simulink model "PID_MOJ"  (R2022b)
settings: Solver=VariableStepAuto  StartTime=0.0  StopTime=10  RelTol=10e-10
values from neighbouring files (symbols this model uses):
  B = 5    [DANE_TRANSMITANCJA.m]
  D = 1    [DANE_TRANSMITANCJA.m]
  g = 9.81    [DANE_TRANSMITANCJA.m]
  J = 0.2    [DANE_TRANSMITANCJA.m]
  k = 700000    [DANE_TRANSMITANCJA.m]
  ke = 2    [DANE_TRANSMITANCJA.m]
  km = 5    [DANE_TRANSMITANCJA.m]
  Kp = 0.6*Kkr*(1-Tp/Tosc)    (= 22.6944444444)    [DANE_TRANSMITANCJA.m]
  L = 0.1    [DANE_TRANSMITANCJA.m]
  m = 100    [DANE_TRANSMITANCJA.m]
  mp = 100    [DANE_TRANSMITANCJA.m]
  r = 0.2    [DANE_TRANSMITANCJA.m]
  R = 0.4    [DANE_TRANSMITANCJA.m]
  Td = Tp*0.125*(Tosc/Tp)^2/(Tosc/Tp-1)    (= 0.271255813953)    [DANE_TRANSMITANCJA.m]
  Ti = Tp*0.5*(Tosc/Tp-1)    (= 1.075)    [DANE_TRANSMITANCJA.m]
  Tp = 0.01    [DANE_TRANSMITANCJA.m]
undefined symbols (not defined in the file or in its folder): Ld, Md
libraries: slpidlib x4, fuzblock x1
settings Model: Creator=ThePi  LastModifiedBy=ThePi

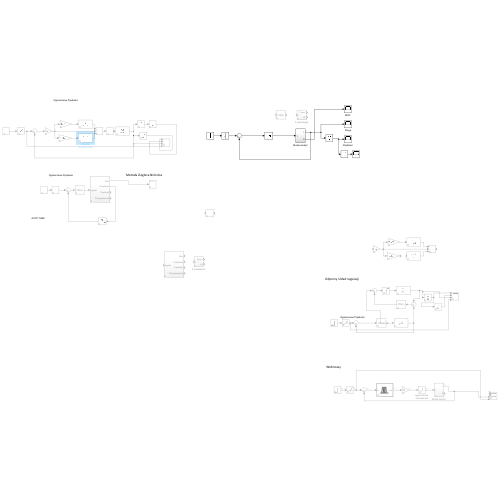
[thumbnail: Simulink's stored preview of the top-level diagram]
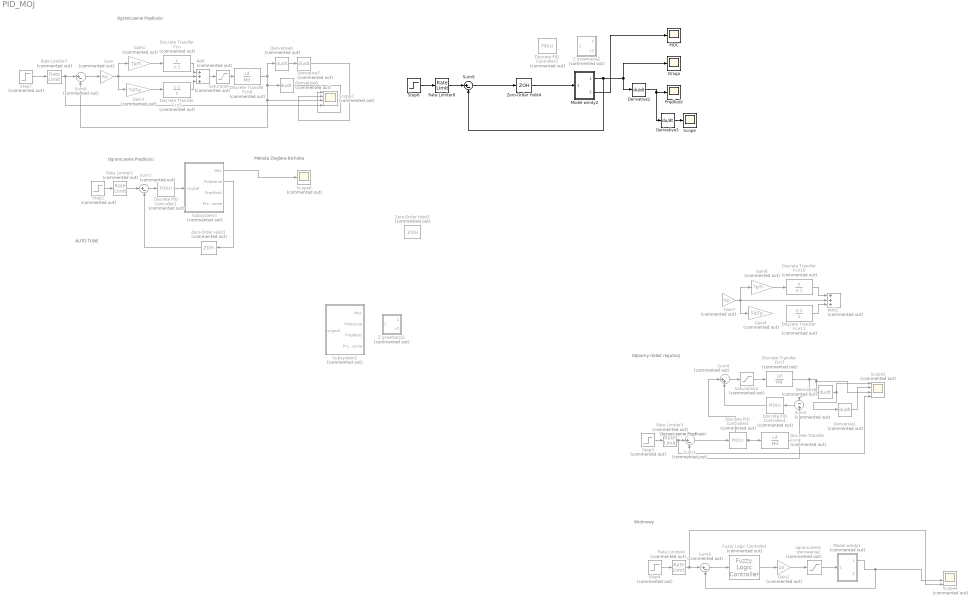
== system PID_MOJ ==
  note: Ograniczenie Prędkości
  note: Metoda Zieglera-Nicholsa
  note: AUTO TUNE
  note: Odporny Układ regulacji
  note: Ograniczenie Prędkości
  note: Ograniczenie Prędkości
  note: WIdmowy
  Add : Sum  Commented=on  Inputs=+++
  Add2 : Sum  Commented=on  Inputs=+++
  Derivative{,1,6..8} (5 alike) : Derivative  Commented=on
  Derivative2 : Derivative
  Derivative3 : Derivative
  Discrete Transfer Fcn : DiscreteTransferFcn  Commented=on  Numerator=[1 0]  Denominator=[1 -1]
  Discrete Transfer Fcn10 : DiscreteTransferFcn  Commented=on  Numerator=[1 0]  Denominator=[1 -1]
  Discrete Transfer Fcn11 : DiscreteTransferFcn  Commented=on  Numerator=[1 -1]  Denominator=[1 0]
  Discrete Transfer Fcn4 : DiscreteTransferFcn  Commented=on  Numerator=Ld  Denominator=Md  SampleTime=Tp
  Discrete Transfer Fcn5 : DiscreteTransferFcn  Commented=on  Numerator=[1 -1]  Denominator=[1 0]
  Discrete Transfer Fcn7 : DiscreteTransferFcn  Commented=on  Numerator=Ld  Denominator=Md  SampleTime=Tp
  Discrete Transfer Fcn8 : DiscreteTransferFcn  Commented=on  Numerator=Ld  Denominator=Md  SampleTime=Tp
  Discrete PID Controller1 : slpidlib/PID Controller  Commented=on  Controller=PID  Form=Ideal  TimeDomain=Discrete-time  UseExternalTs=off  SampleTime=Tp  IntegratorMethod=Forward Euler  FilterMethod=Forward Euler  ControllerParametersSource=internal  P=Kp  I=Ti  UseKiTs=off  D=Td  N=182.532020744323  UseFilter=off  TunerSelectOption=Transfer Function Based (PID Tuner App)  InitialConditionSource=internal  InitialConditionForIntegrator=0  InitialConditionForFilter=0  DifferentiatorICPrevScaledInput=0  ExternalReset=none  TrackingMode=off  Kt=1  LimitOutput=off  SatLimitsSource=internal  UpperSaturationLimit=inf  LowerSaturationLimit=-inf  LinearizeAsGain=off  AntiWindupMode=none  Kb=1  LimitIntegrator=off  UpperIntegratorSaturationLimit=inf  LowerIntegratorSaturationLimit=-inf  POutMin=[]  POutMax=[]  IOutMin=[]  IOutMax=[]  DOutMin=[]  DOutMax=[]  NOutMin=[]  NOutMax=[]  SumOutMin=[]  SumOutMax=[]  SaturationOutMin=[]  SaturationOutMax=[]  PParamMin=[]  PParamMax=[]  IParamMin=[]  IParamMax=[]  DParamMin=[]  DParamMax=[]  NParamMin=[]  NParamMax=[]  KbParamMin=[]  KbParamMax=[]  KtParamMin=[]  KtParamMax=[]  KbOutMin=[]  KbOutMax=[]  KtOutMin=[]  KtOutMax=[]  IntegratorOutMin=[]  IntegratorOutMax=[]  FilterOutMin=[]  FilterOutMax=[]  SumI1OutMin=[]  SumI1OutMax=[]  SumI2OutMin=[]  SumI2OutMax=[]  SumI3OutMin=[]  SumI3OutMax=[]  SumI4OutMin=[]  SumI4OutMax=[]  SumDOutMin=[]  SumDOutMax=[]  DifferentiatorOutMin=[]  DifferentiatorOutMax=[]  FilterDiffOutCoefMin=[]  FilterDiffOutCoefMax=[]  ReciprocalOutMin=[]  ReciprocalOutMax=[]  SumDenOutMin=[]  SumDenOutMax=[]  SumNumOutMin=[]  SumNumOutMax=[]  DivideOutMin=[]  DivideOutMax=[]  UdiffTsProdOutMin=[]  UdiffTsProdOutMax=[]  NTsProdOutMin=[]  NTsProdOutMax=[]  UintegralTsProdOutMin=[]  UintegralTsProdOutMax=[]  UngainTsProdOutMin=[]  UngainTsProdOutMax=[]  ClampingZeroOutDataTypeStr=Inherit: Inherit via back propagation  ClampingZeroOutMin=[]  ClampingZeroOutMax=[]  FilterDenConstantOutDataTypeStr=Inherit: Inherit via back propagation  FilterDenConstantOutMin=[]  FilterDenConstantOutMax=[]  PCopyOutDataTypeStr=Inherit: Inherit via back propagation  PCopyOutMin=[]  PCopyOutMax=[]  NCopyOutDataTypeStr=Inherit: Inherit via back propagation  NCopyOutMin=[]  NCopyOutMax=[]  IntegratorContinuousStateAttributes=''  IntegratorStateMustResolveToSignalObject=off  IntegratorRTWStateStorageClass=Auto  FilterContinuousStateAttributes=''  FilterStateMustResolveToSignalObject=off  FilterRTWStateStorageClass=Auto  ParallelPVariant=Passthrough  IdealPVariant=InternalParameters  IVariant=InternalParameters  DVariant=InternalParameters  IntegratorVariant=Discrete  SatVariant=Disabled  AWVariant=Passthrough  PCopyVariant=Disabled  TRVariant=Disabled  FdbkBlocksVariant=Forward  IdealPFdbkVariant=Disabled  SatFdbkVariant=Disabled  DerivativeFilterVariant=Differentiator  NVariant=Passthrough  NCopyVariant=Disabled_SignalSpec  FilterICVariant=InternalICsDifferentiator  IntegratorICVariant=InternalICs  ExternalResetVariant=Disabled  TRSumVariant=Passthrough  SumFdbkVariant=Disabled  SumVariant=Sum_PID  TsampFilterVariant=InternalTs  TsampNgainVariant=Passthrough  TsampIntegralVariant=Passthrough  ExternalSaturationOutDataTypeStr=Inherit: Same as second input
      settings: LibrarySourceBlock=simulink/Discrete/Discrete PID Controller
  Discrete PID Controller2 : slpidlib/PID Controller  Commented=on  Controller=PID  Form=Ideal  TimeDomain=Discrete-time  UseExternalTs=off  SampleTime=Tp  IntegratorMethod=Forward Euler  FilterMethod=Forward Euler  ControllerParametersSource=internal  P=0.623272871396858  I=0.0120978996964584  UseKiTs=off  D=8.78542633879277  N=15.243341638906  UseFilter=on  TunerSelectOption=Transfer Function Based (PID Tuner App)  InitialConditionSource=internal  InitialConditionForIntegrator=0  InitialConditionForFilter=0  DifferentiatorICPrevScaledInput=0  ExternalReset=none  TrackingMode=off  Kt=1  LimitOutput=off  SatLimitsSource=internal  UpperSaturationLimit=inf  LowerSaturationLimit=-inf  LinearizeAsGain=off  AntiWindupMode=none  Kb=1  LimitIntegrator=off  UpperIntegratorSaturationLimit=inf  LowerIntegratorSaturationLimit=-inf  POutMin=[]  POutMax=[]  IOutMin=[]  IOutMax=[]  DOutMin=[]  DOutMax=[]  NOutMin=[]  NOutMax=[]  SumOutMin=[]  SumOutMax=[]  SaturationOutMin=[]  SaturationOutMax=[]  PParamMin=[]  PParamMax=[]  IParamMin=[]  IParamMax=[]  DParamMin=[]  DParamMax=[]  NParamMin=[]  NParamMax=[]  KbParamMin=[]  KbParamMax=[]  KtParamMin=[]  KtParamMax=[]  KbOutMin=[]  KbOutMax=[]  KtOutMin=[]  KtOutMax=[]  IntegratorOutMin=[]  IntegratorOutMax=[]  FilterOutMin=[]  FilterOutMax=[]  SumI1OutMin=[]  SumI1OutMax=[]  SumI2OutMin=[]  SumI2OutMax=[]  SumI3OutMin=[]  SumI3OutMax=[]  SumI4OutMin=[]  SumI4OutMax=[]  SumDOutMin=[]  SumDOutMax=[]  DifferentiatorOutMin=[]  DifferentiatorOutMax=[]  FilterDiffOutCoefMin=[]  FilterDiffOutCoefMax=[]  ReciprocalOutMin=[]  ReciprocalOutMax=[]  SumDenOutMin=[]  SumDenOutMax=[]  SumNumOutMin=[]  SumNumOutMax=[]  DivideOutMin=[]  DivideOutMax=[]  UdiffTsProdOutMin=[]  UdiffTsProdOutMax=[]  NTsProdOutMin=[]  NTsProdOutMax=[]  UintegralTsProdOutMin=[]  UintegralTsProdOutMax=[]  UngainTsProdOutMin=[]  UngainTsProdOutMax=[]  ClampingZeroOutDataTypeStr=Inherit: Inherit via back propagation  ClampingZeroOutMin=[]  ClampingZeroOutMax=[]  FilterDenConstantOutDataTypeStr=Inherit: Inherit via back propagation  FilterDenConstantOutMin=[]  FilterDenConstantOutMax=[]  PCopyOutDataTypeStr=Inherit: Inherit via back propagation  PCopyOutMin=[]  PCopyOutMax=[]  NCopyOutDataTypeStr=Inherit: Inherit via back propagation  NCopyOutMin=[]  NCopyOutMax=[]  IntegratorContinuousStateAttributes=''  IntegratorStateMustResolveToSignalObject=off  IntegratorRTWStateStorageClass=Auto  FilterContinuousStateAttributes=''  FilterStateMustResolveToSignalObject=off  FilterRTWStateStorageClass=Auto  ParallelPVariant=Passthrough  IdealPVariant=InternalParameters  IVariant=InternalParameters  DVariant=InternalParameters  IntegratorVariant=Discrete  SatVariant=Disabled  AWVariant=Passthrough  PCopyVariant=Disabled  TRVariant=Disabled  FdbkBlocksVariant=Forward  IdealPFdbkVariant=Disabled  SatFdbkVariant=Disabled  DerivativeFilterVariant=ForwardEulerFilter  NVariant=InternalParameters  NCopyVariant=Disabled  FilterICVariant=InternalICsFilter  IntegratorICVariant=InternalICs  ExternalResetVariant=Disabled  TRSumVariant=Passthrough  SumFdbkVariant=Disabled  SumVariant=Sum_PID  TsampFilterVariant=InternalTs  TsampNgainVariant=Passthrough  TsampIntegralVariant=Passthrough  ExternalSaturationOutDataTypeStr=Inherit: Same as second input
      settings: LibrarySourceBlock=simulink/Discrete/Discrete PID Controller
  Discrete PID Controller4 : slpidlib/PID Controller  Commented=on  Controller=PID  Form=Parallel  TimeDomain=Discrete-time  UseExternalTs=off  SampleTime=-1  IntegratorMethod=Forward Euler  FilterMethod=Forward Euler  ControllerParametersSource=internal  P=19.8736932517728  I=4.86889756951287  UseKiTs=off  D=6.56817655006432  N=182.532020744323  UseFilter=off  TunerSelectOption=Transfer Function Based (PID Tuner App)  InitialConditionSource=internal  InitialConditionForIntegrator=0  InitialConditionForFilter=0  DifferentiatorICPrevScaledInput=0  ExternalReset=none  TrackingMode=off  Kt=1  LimitOutput=off  SatLimitsSource=internal  UpperSaturationLimit=inf  LowerSaturationLimit=-inf  LinearizeAsGain=off  AntiWindupMode=none  Kb=1  LimitIntegrator=off  UpperIntegratorSaturationLimit=inf  LowerIntegratorSaturationLimit=-inf  POutMin=[]  POutMax=[]  IOutMin=[]  IOutMax=[]  DOutMin=[]  DOutMax=[]  NOutMin=[]  NOutMax=[]  SumOutMin=[]  SumOutMax=[]  SaturationOutMin=[]  SaturationOutMax=[]  PParamMin=[]  PParamMax=[]  IParamMin=[]  IParamMax=[]  DParamMin=[]  DParamMax=[]  NParamMin=[]  NParamMax=[]  KbParamMin=[]  KbParamMax=[]  KtParamMin=[]  KtParamMax=[]  KbOutMin=[]  KbOutMax=[]  KtOutMin=[]  KtOutMax=[]  IntegratorOutMin=[]  IntegratorOutMax=[]  FilterOutMin=[]  FilterOutMax=[]  SumI1OutMin=[]  SumI1OutMax=[]  SumI2OutMin=[]  SumI2OutMax=[]  SumI3OutMin=[]  SumI3OutMax=[]  SumI4OutMin=[]  SumI4OutMax=[]  SumDOutMin=[]  SumDOutMax=[]  DifferentiatorOutMin=[]  DifferentiatorOutMax=[]  FilterDiffOutCoefMin=[]  FilterDiffOutCoefMax=[]  ReciprocalOutMin=[]  ReciprocalOutMax=[]  SumDenOutMin=[]  SumDenOutMax=[]  SumNumOutMin=[]  SumNumOutMax=[]  DivideOutMin=[]  DivideOutMax=[]  UdiffTsProdOutMin=[]  UdiffTsProdOutMax=[]  NTsProdOutMin=[]  NTsProdOutMax=[]  UintegralTsProdOutMin=[]  UintegralTsProdOutMax=[]  UngainTsProdOutMin=[]  UngainTsProdOutMax=[]  ClampingZeroOutDataTypeStr=Inherit: Inherit via back propagation  ClampingZeroOutMin=[]  ClampingZeroOutMax=[]  FilterDenConstantOutDataTypeStr=Inherit: Inherit via back propagation  FilterDenConstantOutMin=[]  FilterDenConstantOutMax=[]  PCopyOutDataTypeStr=Inherit: Inherit via back propagation  PCopyOutMin=[]  PCopyOutMax=[]  NCopyOutDataTypeStr=Inherit: Inherit via back propagation  NCopyOutMin=[]  NCopyOutMax=[]  IntegratorContinuousStateAttributes=''  IntegratorStateMustResolveToSignalObject=off  IntegratorRTWStateStorageClass=Auto  FilterContinuousStateAttributes=''  FilterStateMustResolveToSignalObject=off  FilterRTWStateStorageClass=Auto  ParallelPVariant=InternalParameters  IdealPVariant=Disabled  IVariant=InternalParameters  DVariant=InternalParameters  IntegratorVariant=Discrete  SatVariant=Disabled  AWVariant=Passthrough  PCopyVariant=Disabled  TRVariant=Disabled  FdbkBlocksVariant=Forward  IdealPFdbkVariant=Disabled  SatFdbkVariant=Disabled  DerivativeFilterVariant=Differentiator  NVariant=Passthrough  NCopyVariant=Disabled_SignalSpec  FilterICVariant=InternalICsDifferentiator  IntegratorICVariant=InternalICs  ExternalResetVariant=Disabled  TRSumVariant=Passthrough  SumFdbkVariant=Disabled  SumVariant=Sum_PID  TsampFilterVariant=InternalTs  TsampNgainVariant=Passthrough  TsampIntegralVariant=Passthrough  ExternalSaturationOutDataTypeStr=Inherit: Same as second input
      settings: LibrarySourceBlock=simulink/Discrete/Discrete PID Controller
  Discrete PID Controller5 : slpidlib/PID Controller  Commented=on  Controller=PID  Form=Ideal  TimeDomain=Discrete-time  UseExternalTs=off  SampleTime=Tp  IntegratorMethod=Forward Euler  FilterMethod=Forward Euler  ControllerParametersSource=internal  P=18.4427572090829  I=0.268340065032812  UseKiTs=off  D=0.559716120813621  N=30.7688755395407  UseFilter=on  TunerSelectOption=Transfer Function Based (PID Tuner App)  InitialConditionSource=internal  InitialConditionForIntegrator=0  InitialConditionForFilter=0  DifferentiatorICPrevScaledInput=0  ExternalReset=none  TrackingMode=off  Kt=1  LimitOutput=off  SatLimitsSource=internal  UpperSaturationLimit=inf  LowerSaturationLimit=-inf  LinearizeAsGain=off  AntiWindupMode=none  Kb=1  LimitIntegrator=off  UpperIntegratorSaturationLimit=inf  LowerIntegratorSaturationLimit=-inf  POutMin=[]  POutMax=[]  IOutMin=[]  IOutMax=[]  DOutMin=[]  DOutMax=[]  NOutMin=[]  NOutMax=[]  SumOutMin=[]  SumOutMax=[]  SaturationOutMin=[]  SaturationOutMax=[]  PParamMin=[]  PParamMax=[]  IParamMin=[]  IParamMax=[]  DParamMin=[]  DParamMax=[]  NParamMin=[]  NParamMax=[]  KbParamMin=[]  KbParamMax=[]  KtParamMin=[]  KtParamMax=[]  KbOutMin=[]  KbOutMax=[]  KtOutMin=[]  KtOutMax=[]  IntegratorOutMin=[]  IntegratorOutMax=[]  FilterOutMin=[]  FilterOutMax=[]  SumI1OutMin=[]  SumI1OutMax=[]  SumI2OutMin=[]  SumI2OutMax=[]  SumI3OutMin=[]  SumI3OutMax=[]  SumI4OutMin=[]  SumI4OutMax=[]  SumDOutMin=[]  SumDOutMax=[]  DifferentiatorOutMin=[]  DifferentiatorOutMax=[]  FilterDiffOutCoefMin=[]  FilterDiffOutCoefMax=[]  ReciprocalOutMin=[]  ReciprocalOutMax=[]  SumDenOutMin=[]  SumDenOutMax=[]  SumNumOutMin=[]  SumNumOutMax=[]  DivideOutMin=[]  DivideOutMax=[]  UdiffTsProdOutMin=[]  UdiffTsProdOutMax=[]  NTsProdOutMin=[]  NTsProdOutMax=[]  UintegralTsProdOutMin=[]  UintegralTsProdOutMax=[]  UngainTsProdOutMin=[]  UngainTsProdOutMax=[]  ClampingZeroOutDataTypeStr=Inherit: Inherit via back propagation  ClampingZeroOutMin=[]  ClampingZeroOutMax=[]  FilterDenConstantOutDataTypeStr=Inherit: Inherit via back propagation  FilterDenConstantOutMin=[]  FilterDenConstantOutMax=[]  PCopyOutDataTypeStr=Inherit: Inherit via back propagation  PCopyOutMin=[]  PCopyOutMax=[]  NCopyOutDataTypeStr=Inherit: Inherit via back propagation  NCopyOutMin=[]  NCopyOutMax=[]  IntegratorContinuousStateAttributes=''  IntegratorStateMustResolveToSignalObject=off  IntegratorRTWStateStorageClass=Auto  FilterContinuousStateAttributes=''  FilterStateMustResolveToSignalObject=off  FilterRTWStateStorageClass=Auto  ParallelPVariant=Passthrough  IdealPVariant=InternalParameters  IVariant=InternalParameters  DVariant=InternalParameters  IntegratorVariant=Discrete  SatVariant=Disabled  AWVariant=Passthrough  PCopyVariant=Disabled  TRVariant=Disabled  FdbkBlocksVariant=Forward  IdealPFdbkVariant=Disabled  SatFdbkVariant=Disabled  DerivativeFilterVariant=ForwardEulerFilter  NVariant=InternalParameters  NCopyVariant=Disabled  FilterICVariant=InternalICsFilter  IntegratorICVariant=InternalICs  ExternalResetVariant=Disabled  TRSumVariant=Passthrough  SumFdbkVariant=Disabled  SumVariant=Sum_PID  TsampFilterVariant=InternalTs  TsampNgainVariant=Passthrough  TsampIntegralVariant=Passthrough  ExternalSaturationOutDataTypeStr=Inherit: Same as second input
      settings: LibrarySourceBlock=simulink/Discrete/Discrete PID Controller
  Droga : Scope
  Fuzzy Logic Controller : fuzblock/Fuzzy Logic  Controller  Commented=on  FIS='uni.fis'  OutputSampleNumber=101  DataType=double  FuzzifiedInputs=off  RuleFiringStrengths=off  RuleOutputs=off  AggregatedOutputs=off  SimulateUsing=Interpreted execution  OutOfRangeInputValueMessage=warning  NoRuleFiredMessage=warning  EmptyOutputFuzzySetMessage=warning
  Gain : Gain  Commented=on  Gain=Kp
  Gain1 : Gain  Commented=on  Gain=Tp/Ti
  Gain2 : Gain  Commented=on  Gain=10
  Gain3 : Gain  Commented=on  Gain=Td/Tp
  Gain7 : Gain  Commented=on  Gain=Kp
  Gain8 : Gain  Commented=on  Gain=Tp/Ti
  Gain9 : Gain  Commented=on  Gain=Td/Tp
  MOC : Scope
  Model windy1 : Subsystem  Commented=on
  Model windy2 : Subsystem
  Prędkość : Scope
  Rate Limiter{1,3..4,7} (4 alike) : RateLimiter  Commented=on  RisingSlewLimit=10  FallingSlewLimit=-10  SampleTimeMode=inherited
  Rate Limiter8 : RateLimiter  RisingSlewLimit=10  FallingSlewLimit=-10  SampleTimeMode=inherited
  Saturation : Saturate  Commented=on  UpperLimit=35  LowerLimit=-35
  Saturation2 : Saturate  Commented=on  UpperLimit=45  LowerLimit=-45
  Scope : Scope
  Scope4 : Scope  Commented=on  NumInputPorts=4
  Scope5 : Scope  Commented=on  NumInputPorts=4
  Scope7 : Scope  Commented=on  NumInputPorts=4
  Scope8 : Scope  Commented=on
  Step{1,3..4,7} (4 alike) : Step  Commented=on  Time=0  After=10  SampleTime=Tp
  Step8 : Step  Time=0  After=10  SampleTime=Tp
  Subsystem2 : Subsystem  Commented=on
  Subsystem3 : Subsystem  Commented=on
  Sum{1,3,6,8} (4 alike) : Sum  Commented=on  Inputs=|+-
  Sum4 : Sum  Commented=on  Inputs=|++
  Sum5 : Sum  Commented=on  Inputs=-+
  Sum9 : Sum  Inputs=|+-
  Z grawitacją1 : Subsystem  Commented=on
  Z grawitacją2 : Subsystem  Commented=on
  Zero-Order Hold1 : ZeroOrderHold  Commented=on  SampleTime=-1
  Zero-Order Hold3 : ZeroOrderHold  Commented=on  SampleTime=Tp
  Zero-Order Hold4 : ZeroOrderHold  SampleTime=Tp
  ograniczenie sterowania2 : Saturate  Commented=on  UpperLimit=45  LowerLimit=-45
  wires:
  Rate Limiter1/1 -> Sum1/1
  Sum1/1 -> Discrete PID Controller1/1
  Discrete PID Controller1/1 -> Subsystem3/1(sygnał)
  Sum3/1 -> Discrete PID Controller5/1
  Discrete PID Controller5/1 -> Sum4/1, Discrete Transfer Fcn4/1
  Discrete Transfer Fcn4/1 -> Sum5/2, Sum3/2
  Step3/1 -> Rate Limiter3/1
  Rate Limiter3/1 -> Scope5/4, Sum3/1
  Discrete PID Controller4/1 -> Sum4/2
  Sum5/1 -> Discrete PID Controller4/1
  Discrete Transfer Fcn7/1 -> Scope5/3, Derivative/1, Sum5/1
  Derivative/1 -> Scope5/1, Derivative1/1
  Derivative1/1 -> Scope5/2
  Sum4/1 -> Saturation2/1
  Sum6/1 -> Fuzzy Logic Controller/1
  Fuzzy Logic Controller/1 -> Gain2/1
  Step4/1 -> Rate Limiter4/1
  Rate Limiter4/1 -> Scope4/4, Sum6/1
  Model windy1/1(Out1) -> Sum6/2, Scope4/3
  ograniczenie sterowania2/1 -> Model windy1/1(In1)
  Gain2/1 -> ograniczenie sterowania2/1
  Step1/1 -> Rate Limiter1/1
  Saturation2/1 -> Discrete Transfer Fcn7/1
  Step7/1 -> Rate Limiter7/1
  Discrete Transfer Fcn8/1 -> Derivative8/1, Scope7/3, Sum8/2, Derivative6/1
  Rate Limiter7/1 -> Scope7/4, Sum8/1
  Sum8/1 -> Gain/1
  Gain/1 -> Gain1/1, Add/2, Gain3/1
  Gain1/1 -> Discrete Transfer Fcn/1
  Gain3/1 -> Discrete Transfer Fcn5/1
  Discrete Transfer Fcn5/1 -> Add/3
  Discrete Transfer Fcn/1 -> Add/1
  Add/1 -> Saturation/1
  Derivative6/1 -> Derivative7/1
  Derivative7/1 -> Scope7/1
  Derivative8/1 -> Scope7/2
  Subsystem3/2(Położenie) -> Zero-Order Hold1/1
  Zero-Order Hold1/1 -> Sum1/2
  Subsystem3/1(Moc) -> Scope8/1
  Rate Limiter8/1 -> Sum9/1
  Step8/1 -> Rate Limiter8/1
  Model windy2/1(Out1) -> Derivative2/1, Droga/1, Sum9/2
  Gain7/1 -> Gain8/1, Add2/2, Gain9/1
  Gain8/1 -> Discrete Transfer Fcn10/1
  Discrete Transfer Fcn11/1 -> Add2/3
  Discrete Transfer Fcn10/1 -> Add2/1
  Zero-Order Hold4/1 -> Model windy2/1(In1)
  Sum9/1 -> Zero-Order Hold4/1
  Saturation/1 -> Discrete Transfer Fcn8/1
  Derivative2/1 -> Derivative3/1, Prędkość/1
  Derivative3/1 -> Scope/1
  Model windy2/2(Out2) -> MOC/1

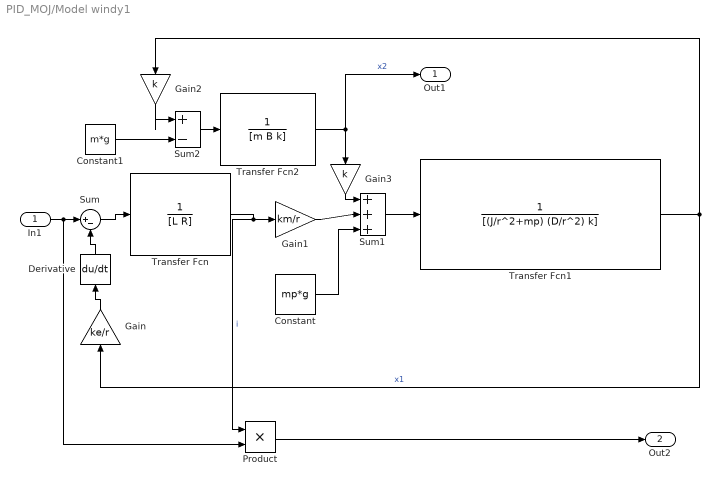
== system PID_MOJ/Model windy1 ==
  In1 : Inport
  Constant : Constant  Value=mp*g
  Constant1 : Constant  Value=m*g
  Derivative : Derivative
  Gain : Gain  Gain=ke/r
  Gain1 : Gain  Gain=km/r
  Gain2 : Gain  Gain=k
  Gain3 : Gain  Gain=k
  Product : Product
  Sum : Sum  Inputs=|+-
  Sum1 : Sum  Inputs=|+++
  Sum2 : Sum  Inputs=|+-
  Transfer Fcn : TransferFcn  Denominator=[L R]
  Transfer Fcn1 : TransferFcn  Denominator=[(J/r^2+mp) (D/r^2) k]
  Transfer Fcn2 : TransferFcn  Denominator=[m B k]
  Out1 : Outport
  Out2 : Outport  Port=2
  wires:
  Gain3/1 -> Sum1/1
  Sum/1 -> Transfer Fcn/1
  Gain/1 -> Derivative/1
  Gain2/1 -> Sum2/1
  Gain1/1 -> Sum1/2
  Derivative/1 -> Sum/2
  Transfer Fcn/1 -> Product/1, Gain1/1  "i"
  Transfer Fcn2/1 -> Out1/1, Gain3/1  "x2"
  Sum2/1 -> Transfer Fcn2/1
  Sum1/1 -> Transfer Fcn1/1
  In1/1 -> Product/2, Sum/1
  Product/1 -> Out2/1
  Transfer Fcn1/1 -> Gain/1, Gain2/1  "x1"
  Constant1/1 -> Sum2/2
  Constant/1 -> Sum1/3

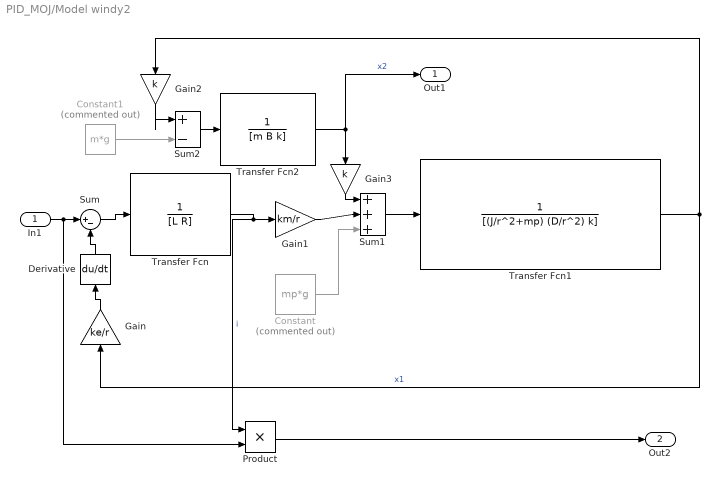
== system PID_MOJ/Model windy2 ==
  In1 : Inport
  Constant : Constant  Commented=on  Value=mp*g
  Constant1 : Constant  Commented=on  Value=m*g
  Derivative : Derivative
  Gain : Gain  Gain=ke/r
  Gain1 : Gain  Gain=km/r
  Gain2 : Gain  Gain=k
  Gain3 : Gain  Gain=k
  Product : Product
  Sum : Sum  Inputs=|+-
  Sum1 : Sum  Inputs=|+++
  Sum2 : Sum  Inputs=|+-
  Transfer Fcn : TransferFcn  Denominator=[L R]
  Transfer Fcn1 : TransferFcn  Denominator=[(J/r^2+mp) (D/r^2) k]
  Transfer Fcn2 : TransferFcn  Denominator=[m B k]
  Out1 : Outport
  Out2 : Outport  Port=2
  wires:
  Constant/1 -> Sum1/3
  Constant1/1 -> Sum2/2
  Transfer Fcn1/1 -> Gain2/1, Gain/1  "x1"
  Product/1 -> Out2/1
  In1/1 -> Sum/1, Product/2
  Sum1/1 -> Transfer Fcn1/1
  Sum2/1 -> Transfer Fcn2/1
  Transfer Fcn2/1 -> Gain3/1, Out1/1  "x2"
  Transfer Fcn/1 -> Gain1/1, Product/1  "i"
  Derivative/1 -> Sum/2
  Gain1/1 -> Sum1/2
  Gain2/1 -> Sum2/1
  Gain/1 -> Derivative/1
  Sum/1 -> Transfer Fcn/1
  Gain3/1 -> Sum1/1

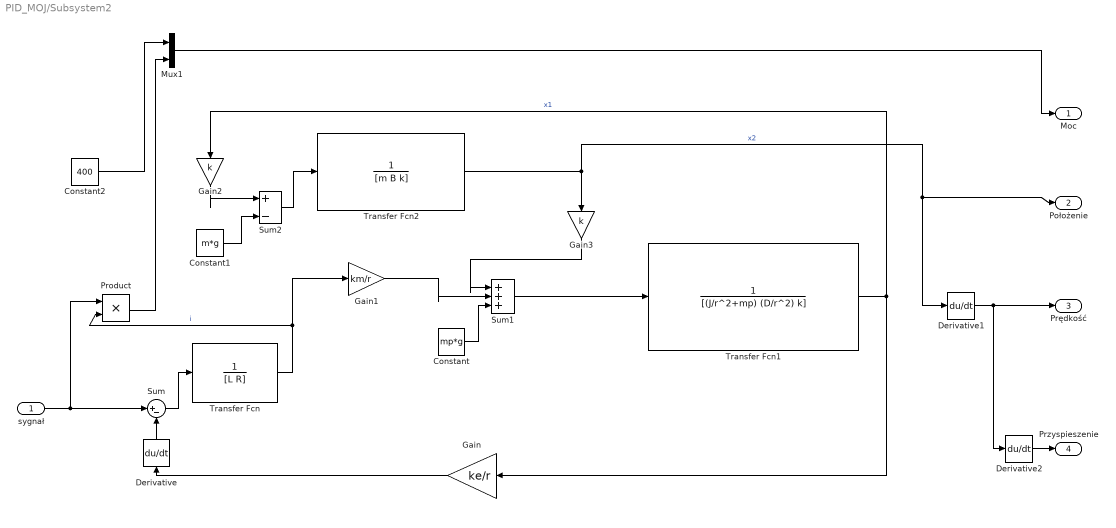
== system PID_MOJ/Subsystem2 ==
  sygnał : Inport  SampleTime=Tp
  Constant : Constant  Value=mp*g
  Constant1 : Constant  Value=m*g
  Constant2 : Constant  Value=400
  Derivative : Derivative
  Derivative1 : Derivative
  Derivative2 : Derivative
  Gain : Gain  Gain=ke/r
  Gain1 : Gain  Gain=km/r
  Gain2 : Gain  Gain=k
  Gain3 : Gain  Gain=k
  Mux1 : Mux  Inputs=2
  Product : Product  RndMeth=Zero
  Sum : Sum  Inputs=|+-
  Sum1 : Sum  Inputs=|+++
  Sum2 : Sum  Inputs=|+-
  Transfer Fcn : TransferFcn  Denominator=[L R]
  Transfer Fcn1 : TransferFcn  Denominator=[(J/r^2+mp) (D/r^2) k]
  Transfer Fcn2 : TransferFcn  Denominator=[m B k]
  Moc : Outport  SampleTime=Tp
  Położenie : Outport  Port=2  SampleTime=Tp
  Prędkość : Outport  Port=3  SampleTime=Tp
  Przyspieszenie : Outport  Port=4  SampleTime=Tp
  wires:
  Gain/1 -> Derivative/1
  Derivative/1 -> Sum/2
  sygnał/1 -> Product/1, Sum/1
  Transfer Fcn/1 -> Gain1/1, Product/2  "i"
  Sum/1 -> Transfer Fcn/1
  Constant/1 -> Sum1/3
  Transfer Fcn1/1 -> Gain/1, Gain2/1  "x1"
  Gain1/1 -> Sum1/2
  Derivative1/1 -> Prędkość/1, Derivative2/1
  Derivative2/1 -> Przyspieszenie/1
  Gain3/1 -> Sum1/1
  Transfer Fcn2/1 -> Gain3/1, Położenie/1, Derivative1/1  "x2"
  Gain2/1 -> Sum2/1
  Constant2/1 -> Mux1/1
  Product/1 -> Mux1/2
  Sum2/1 -> Transfer Fcn2/1
  Mux1/1 -> Moc/1
  Sum1/1 -> Transfer Fcn1/1
  Constant1/1 -> Sum2/2

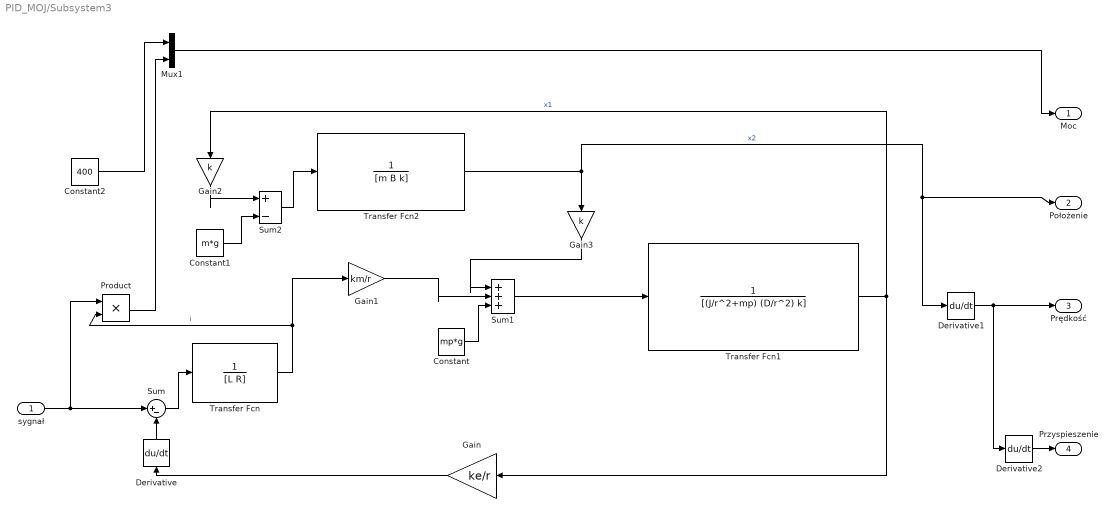
== system PID_MOJ/Subsystem3 ==
  sygnał : Inport  SampleTime=Tp
  Constant : Constant  Value=mp*g
  Constant1 : Constant  Value=m*g
  Constant2 : Constant  Value=400
  Derivative : Derivative
  Derivative1 : Derivative
  Derivative2 : Derivative
  Gain : Gain  Gain=ke/r
  Gain1 : Gain  Gain=km/r
  Gain2 : Gain  Gain=k
  Gain3 : Gain  Gain=k
  Mux1 : Mux  Inputs=2
  Product : Product  RndMeth=Zero
  Sum : Sum  Inputs=|+-
  Sum1 : Sum  Inputs=|+++
  Sum2 : Sum  Inputs=|+-
  Transfer Fcn : TransferFcn  Denominator=[L R]
  Transfer Fcn1 : TransferFcn  Denominator=[(J/r^2+mp) (D/r^2) k]
  Transfer Fcn2 : TransferFcn  Denominator=[m B k]
  Moc : Outport  SampleTime=Tp
  Położenie : Outport  Port=2  SampleTime=Tp
  Prędkość : Outport  Port=3  SampleTime=Tp
  Przyspieszenie : Outport  Port=4  SampleTime=Tp
  wires:
  Gain/1 -> Derivative/1
  Derivative/1 -> Sum/2
  sygnał/1 -> Product/1, Sum/1
  Transfer Fcn/1 -> Gain1/1, Product/2  "i"
  Sum/1 -> Transfer Fcn/1
  Constant/1 -> Sum1/3
  Transfer Fcn1/1 -> Gain/1, Gain2/1  "x1"
  Gain1/1 -> Sum1/2
  Derivative1/1 -> Prędkość/1, Derivative2/1
  Derivative2/1 -> Przyspieszenie/1
  Gain3/1 -> Sum1/1
  Transfer Fcn2/1 -> Gain3/1, Położenie/1, Derivative1/1  "x2"
  Gain2/1 -> Sum2/1
  Constant2/1 -> Mux1/1
  Product/1 -> Mux1/2
  Sum2/1 -> Transfer Fcn2/1
  Mux1/1 -> Moc/1
  Sum1/1 -> Transfer Fcn1/1
  Constant1/1 -> Sum2/2

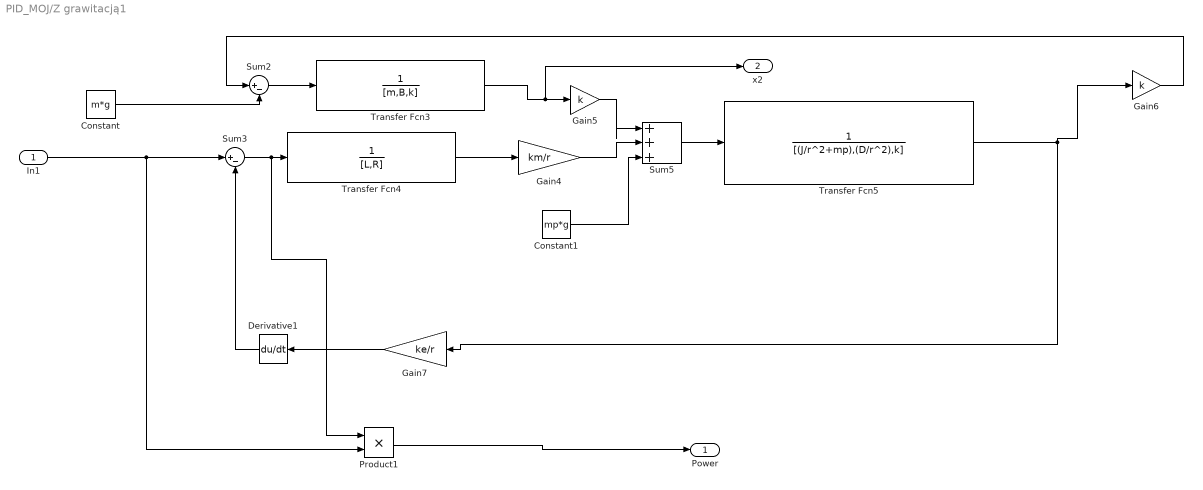
== system PID_MOJ/Z grawitacją1 ==
  In1 : Inport
  Constant : Constant  Value=m*g
  Constant1 : Constant  Value=mp*g
  Derivative1 : Derivative
  Gain4 : Gain  Gain=km/r
  Gain5 : Gain  Gain=k
  Gain6 : Gain  Gain=k
  Gain7 : Gain  Gain=ke/r
  Product1 : Product
  Sum2 : Sum  Inputs=|+-
  Sum3 : Sum  Inputs=|+-
  Sum5 : Sum  Inputs=|+++
  Transfer Fcn3 : TransferFcn  Denominator=[m,B,k]
  Transfer Fcn4 : TransferFcn  Denominator=[L,R]
  Transfer Fcn5 : TransferFcn  Denominator=[(J/r^2+mp),(D/r^2),k]
  Power : Outport
  x2 : Outport  Port=2
  wires:
  Constant/1 -> Sum2/2
  Gain6/1 -> Sum2/1
  Sum2/1 -> Transfer Fcn3/1
  Gain4/1 -> Sum5/2
  Transfer Fcn4/1 -> Gain4/1
  Gain5/1 -> Sum5/1
  Sum5/1 -> Transfer Fcn5/1
  Gain7/1 -> Derivative1/1
  Transfer Fcn3/1 -> Gain5/1, x2/1
  Constant1/1 -> Sum5/3
  In1/1 -> Sum3/1, Product1/2
  Derivative1/1 -> Sum3/2
  Sum3/1 -> Transfer Fcn4/1, Product1/1
  Product1/1 -> Power/1
  Transfer Fcn5/1 -> Gain6/1, Gain7/1

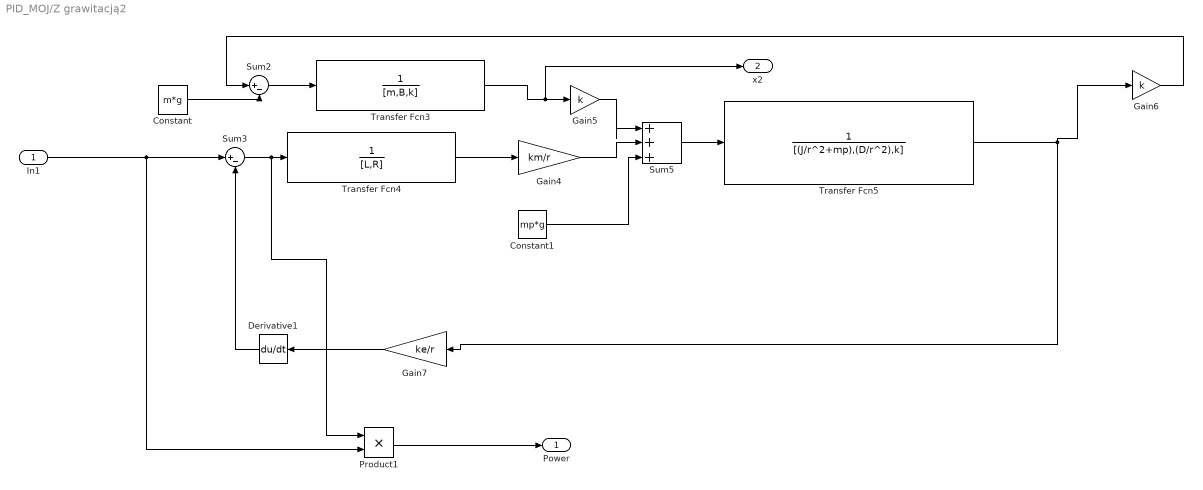
== system PID_MOJ/Z grawitacją2 ==
  In1 : Inport
  Constant : Constant  Value=m*g
  Constant1 : Constant  Value=mp*g
  Derivative1 : Derivative
  Gain4 : Gain  Gain=km/r
  Gain5 : Gain  Gain=k
  Gain6 : Gain  Gain=k
  Gain7 : Gain  Gain=ke/r
  Product1 : Product
  Sum2 : Sum  Inputs=|+-
  Sum3 : Sum  Inputs=|+-
  Sum5 : Sum  Inputs=|+++
  Transfer Fcn3 : TransferFcn  Denominator=[m,B,k]
  Transfer Fcn4 : TransferFcn  Denominator=[L,R]
  Transfer Fcn5 : TransferFcn  Denominator=[(J/r^2+mp),(D/r^2),k]
  Power : Outport
  x2 : Outport  Port=2
  wires:
  Constant/1 -> Sum2/2
  Gain6/1 -> Sum2/1
  Sum2/1 -> Transfer Fcn3/1
  Gain4/1 -> Sum5/2
  Transfer Fcn4/1 -> Gain4/1
  Gain5/1 -> Sum5/1
  Sum5/1 -> Transfer Fcn5/1
  Gain7/1 -> Derivative1/1
  Transfer Fcn3/1 -> Gain5/1, x2/1
  Constant1/1 -> Sum5/3
  In1/1 -> Sum3/1, Product1/2
  Derivative1/1 -> Sum3/2
  Sum3/1 -> Transfer Fcn4/1, Product1/1
  Product1/1 -> Power/1
  Transfer Fcn5/1 -> Gain6/1, Gain7/1
